simulink model "fxpdemo_sine"  (Simulink 5.0)
settings: Solver=FixedStepDiscrete  SolverMode=SingleTasking  StartTime=0.0  StopTime=inf  FixedStep=.01  MaxStep=0.01  RelTol=1e-3  AbsTol=1e-6
libraries: fixpt_lib_4 x4, fixpt_lib_3p1 x1
settings Model: CovMetricSettings=d  MinMaxOverflowLogging=MinMaxAndOverflow  Creator=ciolfi  LastModifiedBy=andyb  ExtModeTrigMode=oneshot  ExtModeArmWhenConnect=off  ExtModeAutoUpdateStatusClock=off  SaveTime=off  SaveOutput=off  LimitDataPoints=off  IntegerOverflowMsg=none  ParameterDowncastMsg=warning  ParameterOverflowMsg=warning  ParameterPrecisionLossMsg=none  RTWInlineParameters=on  RTWOptions="-aEnforceIntegerDowncast=1 -aExtMode=0 -aExtModeTesting=0 -aFoldNonRolledExpr=1 -aForceParamTrailComments=0 -aGenerateComments=1 -aGenerateReport=0 -aIgnoreCustomStorageClasses=1 -aIncDataTypeInIds=0 -aIncHierarchyInIds=0 -aInlineInvariantSignals=1 -aInlinedPrmAccess=\"Literals\" -aLocalBlockOutputs=1 -aLogVarNameModifier=\"rt_\" -aMaxRTWIdLen=31 -aPrefixModelToSubsysFcnNames=1 -aRTWVerbose=1 -aRollThreshold=5 -aShowEliminatedStatements=0"

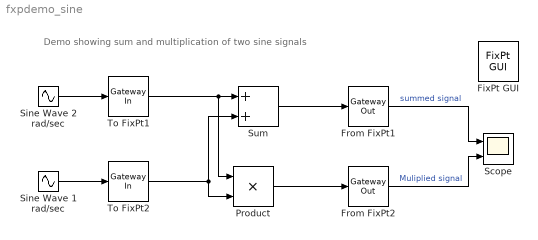
== system fxpdemo_sine ==
  note: Demo showing sum and multiplication of two sine signals
  FixPt GUI : fixpt_lib_3p1/FixPt GUI
  From FixPt1 : fixpt_lib_4/Data Type/Gateway Out  OutRealWorld=Real World Value  OutBuiltInType=double  DoSatur=off
  From FixPt2 : fixpt_lib_4/Data Type/Gateway Out  OutRealWorld=Real World Value  OutBuiltInType=double  DoSatur=off
  Product : Product  ShowAdditionalParam=on  OutDataTypeMode=Specify via dialog  OutScaling=2^-8
  Scope : Scope  NumInputPorts=2
      settings: TickLabels=on  TimeRange=10  YMin=-2.5~-1  YMax=2~1
  Sine Wave 1 rad/sec : Sin  SampleTime=0
  Sine Wave 2 rad/sec : Sin  Frequency=2  SampleTime=0
  Sum : Sum  ShowAdditionalParam=on  OutDataTypeMode=Specify via dialog  OutScaling=2^-2
  To FixPt1 : fixpt_lib_4/Data Type/Gateway In  InRealWorld=Real World Value  OutputDataTypeScalingMode=Specify via dialog  OutDataType=sfix(16)  OutScaling=2^-7  DoSatur=off
  To FixPt2 : fixpt_lib_4/Data Type/Gateway In  InRealWorld=Real World Value  OutputDataTypeScalingMode=Specify via dialog  OutDataType=sfix(16)  OutScaling=2^-6  DoSatur=off
  wires:
  Sine Wave 1 rad/sec/1 -> To FixPt2/1
  Sine Wave 2 rad/sec/1 -> To FixPt1/1
  To FixPt1/1 -> Sum/1, Product/1
  To FixPt2/1 -> Sum/2, Product/2
  From FixPt1/1 -> Scope/1  "summed signal"
  Sum/1 -> From FixPt1/1
  From FixPt2/1 -> Scope/2  "Muliplied signal"
  Product/1 -> From FixPt2/1
